simulink model "HW1no2i"  (R2022b)
settings: Solver=VariableStepAuto  StartTime=0.0  StopTime=10.0  RelTol=1e-3
settings Model: Creator=mluser  LastModifiedBy=Lab417

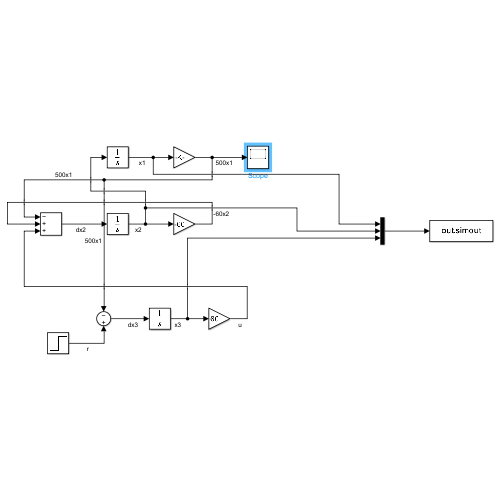
[thumbnail: Simulink's stored preview of the top-level diagram]
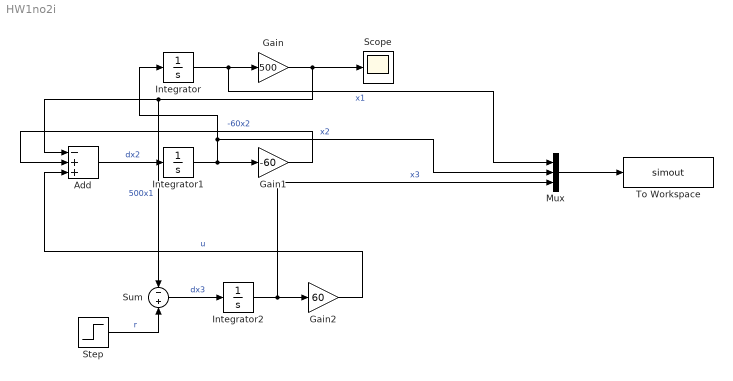
== system HW1no2i ==
  Add : Sum  Inputs=-++
  Gain : Gain  Gain=500
  Gain1 : Gain  Gain=-60
  Gain2 : Gain  Gain=60
  Integrator : Integrator
  Integrator1 : Integrator
  Integrator2 : Integrator
  Mux : Mux  Inputs=3
  Scope : Scope
  Step : Step  Time=0  SampleTime=0
  Sum : Sum  Inputs=-+
  To Workspace : ToWorkspace  VariableName=simout  SaveFormat=Timeseries  SampleTime=-1
  wires:
  Integrator/1 -> Mux/1, Gain/1  "x1"
  Integrator1/1 -> Mux/2, Integrator/1, Gain1/1  "x2"
  Add/1 -> Integrator1/1  "dx2"
  Gain/1 -> Add/1, Sum/1, Scope/1  "500x1"
  Gain1/1 -> Add/2  "-60x2"
  Gain2/1 -> Add/3  "u"
  Integrator2/1 -> Mux/3, Gain2/1  "x3"
  Sum/1 -> Integrator2/1  "dx3"
  Step/1 -> Sum/2  "r"
  Mux/1 -> To Workspace/1
